simulink model "DeepWaySILForSLX_Trailer_2021a_SteerAngle"  (R2021a)
settings: Solver=FixedStepDiscrete  StartTime=0.0  StopTime=inf  FixedStep=0.001  RelTol=1e-3
InitFcn:
  | TargetIP='10.50.192.52';
libraries: simulink x14, slrealtimeutilitieslib x9, dspnetwork x4, aerolibanimutils x1
(part 1 of 2)
settings Model: Tag=normal  Creator=caowancang  LastModifiedBy=mapen
settings DataIOCC: SaveFormat=StructureWithTime
settings OptimizationCC: DefaultParameterBehavior=Inlined  OptimizeBlockIOStorage=off  EnhancedBackFolding=on  PassReuseOutputArgsAs=Individual arguments  ZeroExternalMemoryAtStartup=off  ZeroInternalMemoryAtStartup=off  OptimizeBlockOrder=speed  DifferentSizesBufferReuse=on  EfficientTunableParamExpr=on
settings DebuggingCC: UnderspecifiedInitializationDetection=Classic  ParameterTunabilityLossMsg=error  FrameProcessingCompatibilityMsg=warning  NonCurrentReleaseOperatingPointMsg=warning
settings SFSimCC: MATLABDynamicMemAlloc=off
settings RTWCC: SystemTargetFile=ert.tlc  TemplateMakefile=ert_default_tmf
settings CodeAppCC: ForceParamTrailComments=on  IgnoreCustomStorageClasses=off  OperatorAnnotations=on  SimulinkDataObjDesc=on  SFDataObjDesc=on  InsertBlockDesc=on
settings ERTTargetCC: TargetLangStandard=C99 (ISO)  GenerateSampleERTMain=on  InlinedParameterPlacement=NonHierarchical  ERTCustomFileTemplate=example_file_process.tlc

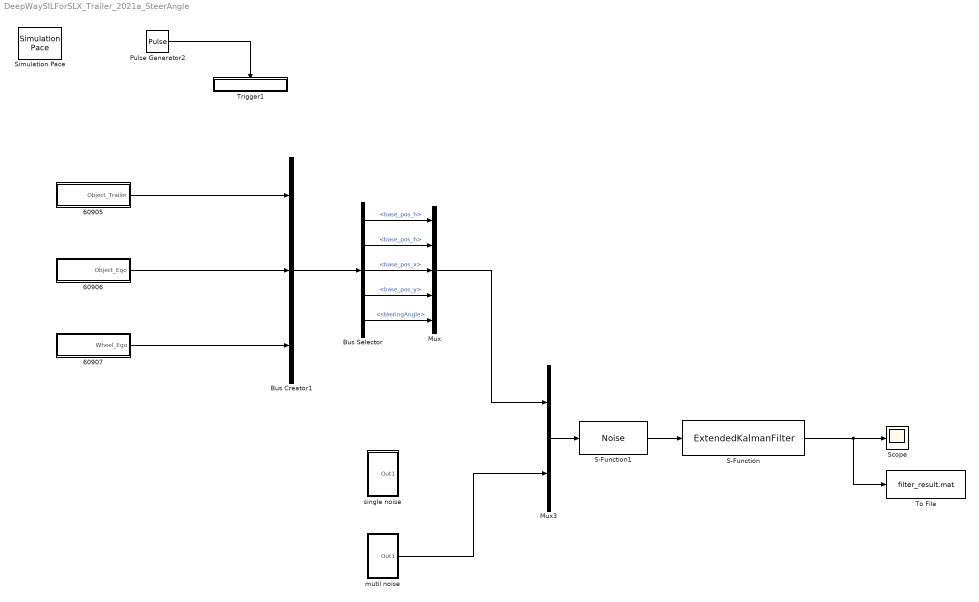
== system DeepWaySILForSLX_Trailer_2021a_SteerAngle ==
  60905 : Subsystem  Description=Modified By caowancang at 2021-11-24 17:03:20.  TreatAsAtomicUnit=on
  60906 : Subsystem  Description=Modified By caowancang at 2021-11-24 17:03:20.  TreatAsAtomicUnit=on
  60907 : Subsystem  Description=Modified By caowancang at 2021-11-24 17:03:20.  TreatAsAtomicUnit=on
  Bus Creator1 : BusCreator  Inputs=3
  Bus Selector : BusSelector  OutputSignals=Object_Ego.Object_Ego.base_pos_h,Object_Trailer.Object_Trailer.base_pos_h,Object_Ego.Object_Ego.base_pos_x,Object_Ego.Object_Ego.base_pos_y,Wheel_Ego.Wheel_Ego.steeringAngle
  Mux : Mux  Inputs=5
  Mux3 : Mux  Inputs=2
  Pulse Generator2 : DiscretePulseGenerator  PulseType=Time based  Period=0.04  PulseWidth=50
  S-Function : S-Function  FunctionName=ExtendedKalmanFilter  SFunctionDeploymentMode=off  EnableBusSupport=off
  S-Function1 : S-Function  FunctionName=Noise  SFunctionDeploymentMode=off  EnableBusSupport=off
  Scope : Scope
  Simulation Pace : aerolibanimutils/Simulation Pace  SimulationPace=1  SleepMode=MATLAB Thread  OutputPaceError=off  SampleTime=-1
      settings: AttributesFormatString=%<SimulationPace> sec/sec
  To File : ToFile  Filename=filter_result.mat  MatrixName=filter_result  SaveFormat=Timeseries
  Trigger1 : Subsystem  Description=Modified By caowancang at 2021-11-26 13:39:19.
  mutil noise : Subsystem
  single noise : Subsystem
  wires:
  60905/1(Object_Trailer) -> Bus Creator1/1
  60906/1(Object_Ego) -> Bus Creator1/2
  Pulse Generator2/1 -> Trigger1/Trigger
  Bus Creator1/1 -> Bus Selector/1
  60907/1(Wheel_Ego) -> Bus Creator1/3
  Bus Selector/1 -> Mux/1  "<base_pos_h>"
  Bus Selector/2 -> Mux/2  "<base_pos_h>"
  Bus Selector/3 -> Mux/3  "<base_pos_x>"
  Bus Selector/4 -> Mux/4  "<base_pos_y>"
  Bus Selector/5 -> Mux/5  "<steeringAngle>"
  Mux/1 -> Mux3/1
  S-Function1/1 -> S-Function/1
  Mux3/1 -> S-Function1/1
  mutil noise/1(Out1) -> Mux3/2
  S-Function/1 -> To File/1, Scope/1

== system DeepWaySILForSLX_Trailer_2021a_SteerAngle/60905 ==
  60905 : Subsystem  Description=Modified By caowancang at 2021-11-18 19:09:14.
  UDP Receive : dspnetwork/UDP Receive  localURL='0.0.0.0'  localPort=60905  remoteURL=TargetIP  remotePort=-1  recvBufferSize=8192  dims=1000  signalDatatype=uint8  isComplex=off  isVarSize=off  showBlockingTime=off  blockingTime=0  sampletime=-1  blockPlatform=[]
  Object_Trailer : Outport  Description=Modified By caowancang at 2021-11-18 18:04:55.
  wires:
  60905/1(Object_Trailer) -> Object_Trailer/1
  UDP Receive/2 -> 60905/2(L)
  UDP Receive/1 -> 60905/1(u)

== system DeepWaySILForSLX_Trailer_2021a_SteerAngle/60906 ==
  60906 : Subsystem  Description=Modified By caowancang at 2021-11-18 19:09:14.
  UDP Receive : dspnetwork/UDP Receive  localURL='0.0.0.0'  localPort=60906  remoteURL=TargetIP  remotePort=-1  recvBufferSize=8192  dims=1000  signalDatatype=uint8  isComplex=off  isVarSize=off  showBlockingTime=off  blockingTime=0  sampletime=-1  blockPlatform=[]
  Object_Ego : Outport  Description=Modified By caowancang at 2021-11-18 18:04:55.
  wires:
  UDP Receive/1 -> 60906/1(u)
  60906/1(Object_Ego) -> Object_Ego/1
  UDP Receive/2 -> 60906/2(L)

== system DeepWaySILForSLX_Trailer_2021a_SteerAngle/60907 ==
  60907 : Subsystem  Description=Modified By caowancang at 2021-11-18 19:09:14.
  UDP Receive : dspnetwork/UDP Receive  localURL='0.0.0.0'  localPort=60907  remoteURL=TargetIP  remotePort=-1  recvBufferSize=8192  dims=1000  signalDatatype=uint8  isComplex=off  isVarSize=off  showBlockingTime=off  blockingTime=0  sampletime=-1  blockPlatform=[]
  Wheel_Ego : Outport  Description=Modified By caowancang at 2021-11-18 18:04:55.
  wires:
  UDP Receive/2 -> 60907/2(L)
  60907/1(Wheel_Ego) -> Wheel_Ego/1
  UDP Receive/1 -> 60907/1(u)

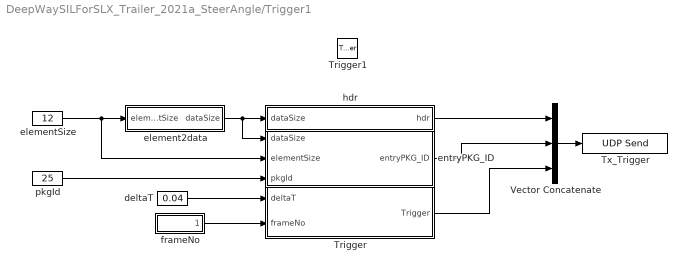
== system DeepWaySILForSLX_Trailer_2021a_SteerAngle/Trigger1 ==
  Trigger1 : TriggerPort  VariantControl=(inherit)
  Trigger : Subsystem  Description=Modified By caowancang at 2021-11-18 02:34:00.
  Tx_Trigger : dspnetwork/UDP Send  remoteURL=TargetIP  remotePort=48191  localURL='0.0.0.0'  localPortSource=Automatically determine  localPort=-1  sendBufferSize=8192  sampletime=-1  blockPlatform=[]  separateLengthPort=0
  Vector Concatenate : Concatenate  NumInputs=3
  deltaT : Constant  Description=Modified By caowancang at 2021-11-29 16:25:47.  Value=0.04
  element2data : Subsystem
  elementSize : Constant  Description=Modified By caowancang at 2021-11-18 02:44:35.  Value=12
  entryPKG_ID : Subsystem  Description=Modified By caowancang at 2021-11-11 11:49:52.
  frameNo : Subsystem
  hdr : Subsystem  Description=Modified By caowancang at 2021-11-11 11:49:52.
  pkgId : Constant  Description=Modified By caowancang at 2021-11-18 02:44:35.  Value=25
  wires:
  entryPKG_ID/1(entryPKG_ID) -> Vector Concatenate/2
  hdr/1(hdr) -> Vector Concatenate/1
  elementSize/1 -> entryPKG_ID/2(elementSize), element2data/1(elementSize)
  element2data/1(dataSize) -> entryPKG_ID/1(dataSize), hdr/1(dataSize)
  Vector Concatenate/1 -> Tx_Trigger/1
  pkgId/1 -> entryPKG_ID/3(pkgId)
  Trigger/1(Trigger) -> Vector Concatenate/3
  deltaT/1 -> Trigger/1(deltaT)
  frameNo/1(frameNo) -> Trigger/2(frameNo)

== system DeepWaySILForSLX_Trailer_2021a_SteerAngle/mutil noise ==
  Mux2 : Mux  Inputs=5
  trailer heading noise : simulink/Sources/Band-Limited White Noise  Cov=[0.05 * 0.05 * 0.1]  Ts=0.1  seed=[23341]
  trator heading noise : simulink/Sources/Band-Limited White Noise  Cov=[0.0 * 0.0 * 0.1]  Ts=0.1  seed=[23341]
  trator steer angle noise : simulink/Sources/Band-Limited White Noise  Cov=[0.00 * 0.00 * 0.1]  Ts=0.1  seed=[23341]
  trator xy noise : simulink/Sources/Band-Limited White Noise  Cov=[0.2 * 0.2 * 0.1]  Ts=0.1  seed=[23341]
  Out1 : Outport
  wires:
  trailer heading noise/1 -> Mux2/2
  trator xy noise/1 -> Mux2/4, Mux2/3
  trator heading noise/1 -> Mux2/1
  Mux2/1 -> Out1/1
  trator steer angle noise/1 -> Mux2/5

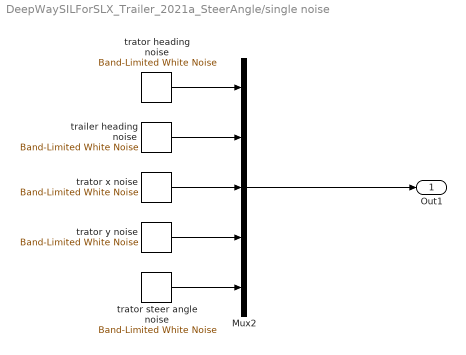
== system DeepWaySILForSLX_Trailer_2021a_SteerAngle/single noise ==
  Mux2 : Mux  Inputs=5
  trailer heading noise : simulink/Sources/Band-Limited White Noise  Cov=[0.05 * 0.05 * 0.1]  Ts=0.1  seed=[23341]
  trator heading noise : simulink/Sources/Band-Limited White Noise  Cov=[0.0 * 0.0 * 0.1]  Ts=0.1  seed=[23341]
  trator steer angle noise : simulink/Sources/Band-Limited White Noise  Cov=[0.0 * 0.0 * 0.1]  Ts=0.1  seed=[23341]
  trator x noise : simulink/Sources/Band-Limited White Noise  Cov=[0.0 * 0.0 * 0.1]  Ts=0.1  seed=[23341]
  trator y noise : simulink/Sources/Band-Limited White Noise  Cov=[0.0 * 0.0 * 0.1]  Ts=0.1  seed=[23341]
  Out1 : Outport
  wires:
  trator y noise/1 -> Mux2/4
  trailer heading noise/1 -> Mux2/2
  trator x noise/1 -> Mux2/3
  trator heading noise/1 -> Mux2/1
  Mux2/1 -> Out1/1
  trator steer angle noise/1 -> Mux2/5

== system DeepWaySILForSLX_Trailer_2021a_SteerAngle/60905/60905 ==
  u : Inport  Description=Modified By caowancang at 2021-11-18 18:43:09.
  L : Inport  Description=Modified By caowancang at 2021-11-18 18:49:26.  Port=2
  98 : Subsystem  Description=Modified By caowancang at 2021-11-18 18:43:09.  TreatAsAtomicUnit=on
  Compare To Constant1 : simulink/Logic and Bit Operations/Compare To Constant  relop===  const=280  OutDataTypeStr=boolean
  Switch Case1 : SwitchCase  CaseConditions={98}  ShowDefaultCase=off
  trigger : Subsystem
  Object_Trailer : Outport  Description=Modified By caowancang at 2021-11-18 18:43:09.
  wires:
  98/1(Object_Trailer) -> Object_Trailer/1
  L/1 -> Compare To Constant1/1
  trigger/1(pkgId) -> Switch Case1/1
  u/1 -> trigger/1(u), 98/1(u)
  Switch Case1/1 -> 98/Action
  Compare To Constant1/1 -> trigger/Trigger

== system DeepWaySILForSLX_Trailer_2021a_SteerAngle/60906/60906 ==
  u : Inport  Description=Modified By caowancang at 2021-11-18 18:43:09.
  L : Inport  Description=Modified By caowancang at 2021-11-18 18:49:26.  Port=2
  97 : Subsystem  Description=Modified By caowancang at 2021-11-18 18:43:09.  TreatAsAtomicUnit=on
  Compare To Constant1 : simulink/Logic and Bit Operations/Compare To Constant  relop===  const=280  OutDataTypeStr=boolean
  Switch Case1 : SwitchCase  CaseConditions={97}  ShowDefaultCase=off
  trigger : Subsystem
  Object_Ego : Outport  Description=Modified By caowancang at 2021-11-18 18:43:09.
  wires:
  97/1(Object_Ego) -> Object_Ego/1
  L/1 -> Compare To Constant1/1
  trigger/1(pkgId) -> Switch Case1/1
  u/1 -> trigger/1(u), 97/1(u)
  Switch Case1/1 -> 97/Action
  Compare To Constant1/1 -> trigger/Trigger

== system DeepWaySILForSLX_Trailer_2021a_SteerAngle/60907/60907 ==
  u : Inport  Description=Modified By caowancang at 2021-11-18 18:43:09.
  L : Inport  Description=Modified By caowancang at 2021-11-18 18:49:26.  Port=2
  99 : Subsystem  Description=Modified By caowancang at 2021-11-18 18:43:09.  TreatAsAtomicUnit=on
  Compare To Constant1 : simulink/Logic and Bit Operations/Compare To Constant  relop===  const=116  OutDataTypeStr=boolean
  Switch Case1 : SwitchCase  CaseConditions={99}  ShowDefaultCase=off
  trigger : Subsystem
  Wheel_Ego : Outport  Description=Modified By caowancang at 2021-11-18 18:43:09.
  wires:
  Compare To Constant1/1 -> trigger/Trigger
  Switch Case1/1 -> 99/Action
  u/1 -> 99/1(u), trigger/1(u)
  trigger/1(pkgId) -> Switch Case1/1
  L/1 -> Compare To Constant1/1
  99/1(Wheel_Ego) -> Wheel_Ego/1

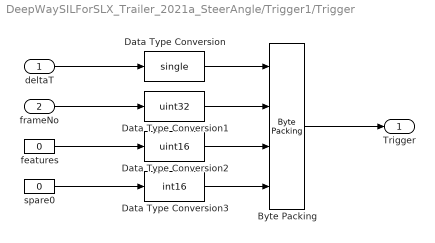
== system DeepWaySILForSLX_Trailer_2021a_SteerAngle/Trigger1/Trigger ==
  deltaT : Inport  Description=Modified By caowancang at 2021-11-18 02:33:49.
  frameNo : Inport  Description=Modified By caowancang at 2021-11-18 02:33:49.  Port=2
  Byte Packing : slrealtimeutilitieslib/Byte Packing  MaskPackedDataType=uint8  MaskUnpackedDataTypes={'single','uint32','uint16','int16'}  MaskAlignment=1
  Data Type Conversion : DataTypeConversion  OutDataTypeStr=single
  Data Type Conversion1 : DataTypeConversion  OutDataTypeStr=uint32
  Data Type Conversion2 : DataTypeConversion  OutDataTypeStr=uint16
  Data Type Conversion3 : DataTypeConversion  OutDataTypeStr=int16
  features : Constant  Description=Modified By caowancang at 2021-11-18 02:33:49.  Value=0
  spare0 : Constant  Description=Modified By caowancang at 2021-11-18 02:33:49.  Value=0
  Trigger : Outport  Description=Modified By caowancang at 2021-11-18 02:33:49.
  wires:
  Data Type Conversion3/1 -> Byte Packing/4
  Data Type Conversion2/1 -> Byte Packing/3
  Data Type Conversion1/1 -> Byte Packing/2
  Data Type Conversion/1 -> Byte Packing/1
  Byte Packing/1 -> Trigger/1
  spare0/1 -> Data Type Conversion3/1
  features/1 -> Data Type Conversion2/1
  frameNo/1 -> Data Type Conversion1/1
  deltaT/1 -> Data Type Conversion/1

== system DeepWaySILForSLX_Trailer_2021a_SteerAngle/Trigger1/element2data ==
  elementSize : Inport  Description=Modified By caowancang at 2021-11-18 02:05:38.
  Constant : Constant  Description=Modified By caowancang at 2021-11-18 02:05:38.
  Product : Product
  dataSize : Outport  Description=Modified By caowancang at 2021-11-18 02:05:38.
  wires:
  Constant/1 -> Product/2
  Product/1 -> dataSize/1
  elementSize/1 -> Product/1

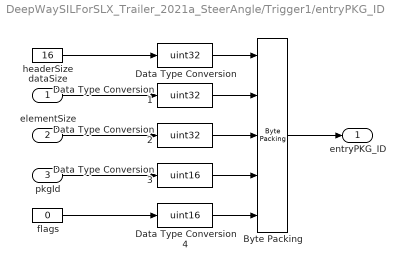
== system DeepWaySILForSLX_Trailer_2021a_SteerAngle/Trigger1/entryPKG_ID ==
  dataSize : Inport  Description=Modified By caowancang at 2021-11-18 02:15:00.
  elementSize : Inport  Description=Modified By caowancang at 2021-11-18 02:15:00.  Port=2
  pkgId : Inport  Description=Modified By caowancang at 2021-11-18 02:15:00.  Port=3
  Byte Packing : slrealtimeutilitieslib/Byte Packing  MaskPackedDataType=uint8  MaskUnpackedDataTypes={'uint32','uint32','uint32','uint16','uint16'}  MaskAlignment=1
  Data Type Conversion : DataTypeConversion  OutDataTypeStr=uint32
  Data Type Conversion1 : DataTypeConversion  OutDataTypeStr=uint32
  Data Type Conversion2 : DataTypeConversion  OutDataTypeStr=uint32
  Data Type Conversion3 : DataTypeConversion  OutDataTypeStr=uint16
  Data Type Conversion4 : DataTypeConversion  OutDataTypeStr=uint16
  flags : Constant  Description=Modified By caowancang at 2021-11-11 11:27:23.  Value=0
  headerSize : Constant  Description=Modified By caowancang at 2021-11-11 11:27:23.  Value=16
  entryPKG_ID : Outport  Description=Modified By caowancang at 2021-11-18 02:24:34.
  wires:
  Data Type Conversion4/1 -> Byte Packing/5
  Data Type Conversion3/1 -> Byte Packing/4
  Data Type Conversion2/1 -> Byte Packing/3
  Data Type Conversion1/1 -> Byte Packing/2
  Data Type Conversion/1 -> Byte Packing/1
  Byte Packing/1 -> entryPKG_ID/1
  headerSize/1 -> Data Type Conversion/1
  dataSize/1 -> Data Type Conversion1/1
  elementSize/1 -> Data Type Conversion2/1
  pkgId/1 -> Data Type Conversion3/1
  flags/1 -> Data Type Conversion4/1

== system DeepWaySILForSLX_Trailer_2021a_SteerAngle/Trigger1/frameNo ==
  Add : Sum
  Compare To Constant : simulink/Logic and Bit Operations/Compare To Constant  relop=>  const=65535  OutDataTypeStr=boolean
  Constant4 : Constant  Description=Modified By caowancang at 2021-11-18 02:07:28.  OutDataTypeStr=uint32
  Switch : Switch  Criteria=u2 ~= 0
  Unit Delay : UnitDelay  SampleTime=-1  HasFrameUpgradeWarning=on
  frameNo : Outport  Description=Modified By caowancang at 2021-11-18 02:07:28.
  wires:
  Compare To Constant/1 -> Switch/2
  Add/1 -> Compare To Constant/1, Switch/3
  Constant4/1 -> Switch/1, Add/1
  Switch/1 -> frameNo/1, Unit Delay/1
  Unit Delay/1 -> Add/2

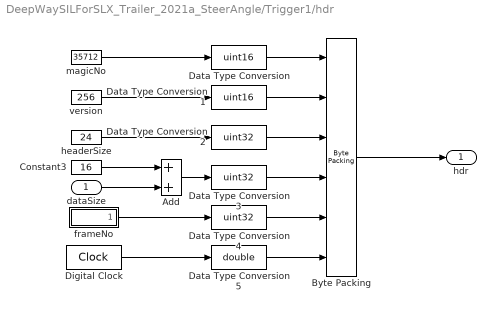
== system DeepWaySILForSLX_Trailer_2021a_SteerAngle/Trigger1/hdr ==
  dataSize : Inport  Description=Modified By caowancang at 2021-11-18 02:12:15.
  Add : Sum
  Byte Packing : slrealtimeutilitieslib/Byte Packing  MaskPackedDataType=uint8  MaskUnpackedDataTypes={'uint16','uint16','uint32','uint32','uint32','double'}  MaskAlignment=1
  Constant3 : Constant  Description=Modified By caowancang at 2021-11-11 11:27:23.  Value=16
  Data Type Conversion : DataTypeConversion  OutDataTypeStr=uint16
  Data Type Conversion1 : DataTypeConversion  OutDataTypeStr=uint16
  Data Type Conversion2 : DataTypeConversion  OutDataTypeStr=uint32
  Data Type Conversion3 : DataTypeConversion  OutDataTypeStr=uint32
  Data Type Conversion4 : DataTypeConversion  OutDataTypeStr=uint32
  Data Type Conversion5 : DataTypeConversion  OutDataTypeStr=double
  Digital Clock : DigitalClock  SampleTime=-1
  frameNo : Subsystem
  headerSize : Constant  Description=Modified By caowancang at 2021-11-11 11:27:23.  Value=24
  magicNo : Constant  Description=Modified By caowancang at 2021-11-11 11:27:23.  Value=35712
  version : Constant  Description=Modified By caowancang at 2021-11-11 11:27:23.  Value=256
  hdr : Outport
  wires:
  Byte Packing/1 -> hdr/1
  Constant3/1 -> Add/1
  Add/1 -> Data Type Conversion3/1
  dataSize/1 -> Add/2
  frameNo/1(frameNo) -> Data Type Conversion4/1
  Digital Clock/1 -> Data Type Conversion5/1
  Data Type Conversion5/1 -> Byte Packing/6
  Data Type Conversion4/1 -> Byte Packing/5
  Data Type Conversion3/1 -> Byte Packing/4
  headerSize/1 -> Data Type Conversion2/1
  Data Type Conversion2/1 -> Byte Packing/3
  version/1 -> Data Type Conversion1/1
  Data Type Conversion1/1 -> Byte Packing/2
  magicNo/1 -> Data Type Conversion/1
  Data Type Conversion/1 -> Byte Packing/1

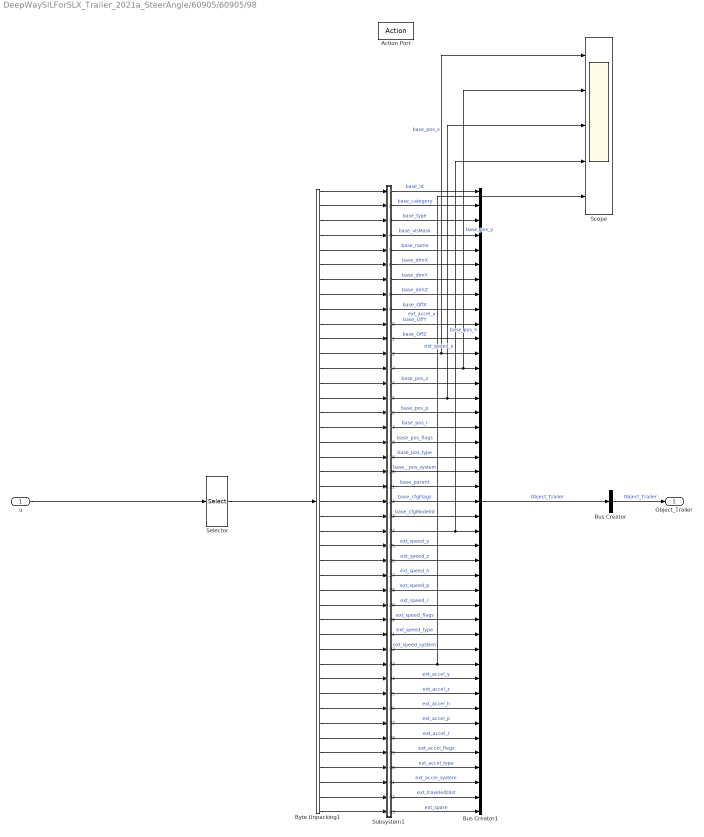
== system DeepWaySILForSLX_Trailer_2021a_SteerAngle/60905/60905/98 ==
  u : Inport  Description=Modified By caowancang at 2021-11-18 14:03:56.
  Action Port : ActionPort  ActionPortLabel=case [ 98 ]:
  Bus Creator : BusCreator  Inputs=1
  Bus Creator1 : BusCreator  Inputs=43
  Byte Unpacking1 : slrealtimeutilitieslib/Byte Unpacking  MaskUnpackedDataTypes={'uint32','uint8','uint8','uint16','uint8','single','single','single','single','single','single','double','double','double','single','single','single','uint8','uint8','uint16','uint32','uint16','int16','double','double','double','single','single','single','uint8','uint8','uint16','double','double','double','single','single','single','uint8','uint8','uint16','single','uint32'}  MaskUnpackedDataSizes={[1],[1],[1],[1],[32],[1],[1],[1],[1],[1],[1],[1],[1],[1],[1],[1],[1],[1],[1],[1],[1],[1],[1],[1],[1],[1],[1],[1],[1],[1],[1],[1],[1],[1],[1],[1],[1],[1],[1],[1],[1],[1],[3]}  MaskAlignment=1
      settings: SourceProductBaseCode=XP
  Scope : Scope  NumInputPorts=5
  Selector : Selector  InputPortWidth=1000  IndexOptions=Starting index (dialog)  Indices=57  OutputSizes=208
  Subsystem1 : Subsystem
  Object_Trailer : Outport  Description=Modified By caowancang at 2021-11-18 14:03:56.
  wires:
  Bus Creator1/1 -> Bus Creator/1  "Object_Trailer"
  Selector/1 -> Byte Unpacking1/1
  u/1 -> Selector/1
  Byte Unpacking1/1 -> Subsystem1/1(In1)
  Byte Unpacking1/2 -> Subsystem1/2(In2)
  Byte Unpacking1/3 -> Subsystem1/3(In3)
  Byte Unpacking1/4 -> Subsystem1/4(In4)
  Byte Unpacking1/5 -> Subsystem1/5(In5)
  Byte Unpacking1/6 -> Subsystem1/6(In6)
  Byte Unpacking1/7 -> Subsystem1/7(In7)
  Byte Unpacking1/8 -> Subsystem1/8(In8)
  Byte Unpacking1/9 -> Subsystem1/9(In9)
  Byte Unpacking1/10 -> Subsystem1/10(In10)
  Byte Unpacking1/11 -> Subsystem1/11(In11)
  Byte Unpacking1/12 -> Subsystem1/12(In12)
  Byte Unpacking1/13 -> Subsystem1/13(In13)
  Byte Unpacking1/14 -> Subsystem1/14(In14)
  Byte Unpacking1/15 -> Subsystem1/15(In15)
  Byte Unpacking1/16 -> Subsystem1/16(In16)
  Byte Unpacking1/17 -> Subsystem1/17(In17)
  Byte Unpacking1/18 -> Subsystem1/18(In18)
  Byte Unpacking1/19 -> Subsystem1/19(In19)
  Byte Unpacking1/20 -> Subsystem1/20(In20)
  Byte Unpacking1/21 -> Subsystem1/21(In21)
  Byte Unpacking1/22 -> Subsystem1/22(In22)
  Byte Unpacking1/23 -> Subsystem1/23(In23)
  Byte Unpacking1/24 -> Subsystem1/24(In24)
  Byte Unpacking1/25 -> Subsystem1/25(In25)
  Byte Unpacking1/26 -> Subsystem1/26(In26)
  Byte Unpacking1/27 -> Subsystem1/27(In27)
  Byte Unpacking1/28 -> Subsystem1/28(In28)
  Byte Unpacking1/29 -> Subsystem1/29(In29)
  Byte Unpacking1/30 -> Subsystem1/30(In30)
  Byte Unpacking1/31 -> Subsystem1/31(In31)
  Byte Unpacking1/32 -> Subsystem1/32(In32)
  Byte Unpacking1/33 -> Subsystem1/33(In33)
  Byte Unpacking1/34 -> Subsystem1/34(In34)
  Byte Unpacking1/35 -> Subsystem1/35(In35)
  Byte Unpacking1/36 -> Subsystem1/36(In36)
  Byte Unpacking1/37 -> Subsystem1/37(In37)
  Byte Unpacking1/38 -> Subsystem1/38(In38)
  Byte Unpacking1/39 -> Subsystem1/39(In39)
  Byte Unpacking1/40 -> Subsystem1/40(In40)
  Byte Unpacking1/41 -> Subsystem1/41(In41)
  Byte Unpacking1/42 -> Subsystem1/42(In42)
  Byte Unpacking1/43 -> Subsystem1/43(In43)
  Subsystem1/1(base_id) -> Bus Creator1/1  "base_id"
  Subsystem1/2(category) -> Bus Creator1/2  "base_category"
  Subsystem1/3(type) -> Bus Creator1/3  "base_type"
  Subsystem1/4(visMask) -> Bus Creator1/4  "base_visMask"
  Subsystem1/5(name) -> Bus Creator1/5  "base_name"
  Subsystem1/6(dimX) -> Bus Creator1/6  "base_dimX"
  Subsystem1/7(dimY) -> Bus Creator1/7  "base_dimY"
  Subsystem1/8(dimZ) -> Bus Creator1/8  "base_dimZ"
  Subsystem1/9(OffX) -> Bus Creator1/9  "base_OffX"
  Subsystem1/10(OffY) -> Bus Creator1/10  "base_OffY"
  Subsystem1/11(OffZ) -> Bus Creator1/11  "base_OffZ"
  Subsystem1/12(pos_x) -> Scope/1, Bus Creator1/12  "base_pos_x"
  Subsystem1/13(pos_y) -> Scope/2, Bus Creator1/13  "base_pos_y"
  Subsystem1/14(pos_z) -> Bus Creator1/14  "base_pos_z"
  Subsystem1/15(pos_h) -> Scope/3, Bus Creator1/15  "base_pos_h"
  Subsystem1/16(pos_p) -> Bus Creator1/16  "base_pos_p"
  Subsystem1/17(pos_r) -> Bus Creator1/17  "base_pos_r"
  Subsystem1/18(flags) -> Bus Creator1/18  "base_pos_flags"
  Subsystem1/19(type1) -> Bus Creator1/19  "base_pos_type"
  Subsystem1/20(system) -> Bus Creator1/20  "base__pos_system"
  Subsystem1/21(parent) -> Bus Creator1/21  "base_parent"
  Subsystem1/22(cfgFlags) -> Bus Creator1/22  "base_cfgFlags"
  Subsystem1/23(cfgModelId) -> Bus Creator1/23  "base_cfgModelId"
  Subsystem1/24(speed_x) -> Scope/4, Bus Creator1/24  "ext_speed_x"
  Subsystem1/25(speed_y) -> Bus Creator1/25  "ext_speed_y"
  Subsystem1/26(speed_z) -> Bus Creator1/26  "ext_speed_z"
  Subsystem1/27(speed_h) -> Bus Creator1/27  "ext_speed_h"
  Subsystem1/28(speed_p) -> Bus Creator1/28  "ext_speed_p"
  Subsystem1/29(speed_r) -> Bus Creator1/29  "ext_speed_r"
  Subsystem1/30(flags2) -> Bus Creator1/30  "ext_speed_flags"
  Subsystem1/31(type3) -> Bus Creator1/31  "ext_speed_type"
  Subsystem1/32(system2) -> Bus Creator1/32  "ext_speed_system"
  Subsystem1/33(accel_x) -> Scope/5, Bus Creator1/33  "ext_accel_x"
  Subsystem1/34(accel_y) -> Bus Creator1/34  "ext_accel_y"
  Subsystem1/35(accel_z) -> Bus Creator1/35  "ext_accel_z"
  Subsystem1/36(accel_h) -> Bus Creator1/36  "ext_accel_h"
  Subsystem1/37(accel_p) -> Bus Creator1/37  "ext_accel_p"
  Subsystem1/38(accel_r) -> Bus Creator1/38  "ext_accel_r"
  Subsystem1/39(flags1) -> Bus Creator1/39  "ext_accel_flags"
  Subsystem1/40(type2) -> Bus Creator1/40  "ext_accel_type"
  Subsystem1/41(system1) -> Bus Creator1/41  "ext_accel_system"
  Subsystem1/42(traveledDist) -> Bus Creator1/42  "ext_traveledDist"
  Subsystem1/43(spare_1) -> Bus Creator1/43  "ext_spare"
  Bus Creator/1 -> Object_Trailer/1  "Object_Trailer"

== system DeepWaySILForSLX_Trailer_2021a_SteerAngle/60905/60905/trigger ==
  u : Inport  Description=Modified By caowancang at 2021-11-18 18:42:51.
  Trigger : TriggerPort  VariantControl=(inherit)
  Byte Unpacking : slrealtimeutilitieslib/Byte Unpacking  MaskUnpackedDataTypes={'uint16'}  MaskUnpackedDataSizes={[1]}  MaskAlignment=1
      settings: SourceProductBaseCode=XP
  Selector : Selector  InputPortWidth=1000  IndexOptions=Starting index (dialog)  Indices=53  OutputSizes=2
  pkgId : Outport  Description=Modified By caowancang at 2021-11-18 18:42:51.
  wires:
  Selector/1 -> Byte Unpacking/1
  u/1 -> Selector/1
  Byte Unpacking/1 -> pkgId/1  "pkgId"

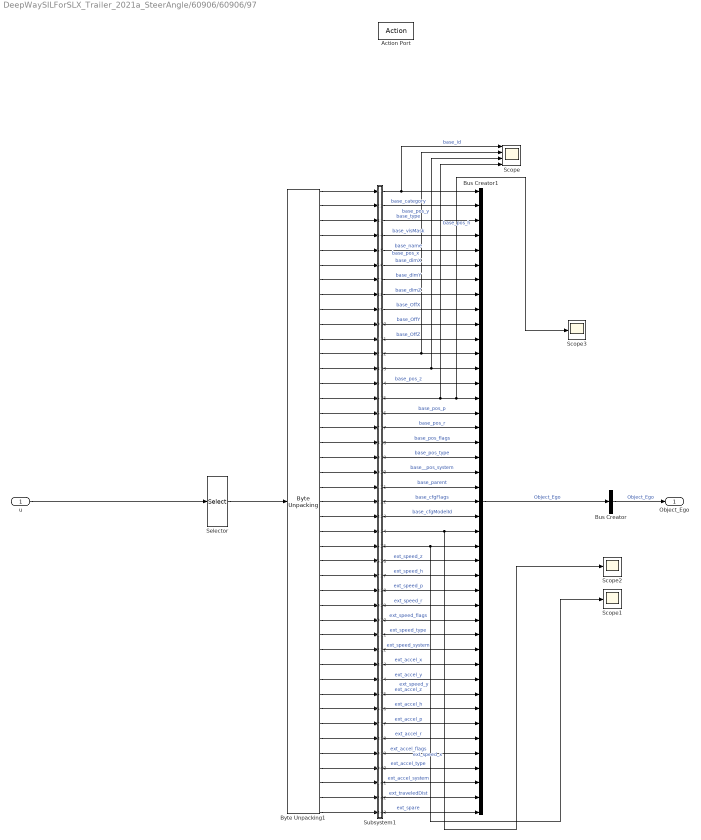
== system DeepWaySILForSLX_Trailer_2021a_SteerAngle/60906/60906/97 ==
  u : Inport  Description=Modified By caowancang at 2021-11-18 14:03:56.
  Action Port : ActionPort  ActionPortLabel=case [ 97 ]:
  Bus Creator : BusCreator  Inputs=1
  Bus Creator1 : BusCreator  Inputs=43
  Byte Unpacking1 : slrealtimeutilitieslib/Byte Unpacking  MaskUnpackedDataTypes={'uint32','uint8','uint8','uint16','uint8','single','single','single','single','single','single','double','double','double','single','single','single','uint8','uint8','uint16','uint32','uint16','int16','double','double','double','single','single','single','uint8','uint8','uint16','double','double','double','single','single','single','uint8','uint8','uint16','single','uint32'}  MaskUnpackedDataSizes={[1],[1],[1],[1],[32],[1],[1],[1],[1],[1],[1],[1],[1],[1],[1],[1],[1],[1],[1],[1],[1],[1],[1],[1],[1],[1],[1],[1],[1],[1],[1],[1],[1],[1],[1],[1],[1],[1],[1],[1],[1],[1],[3]}  MaskAlignment=1
      settings: SourceProductBaseCode=XP
  Scope : Scope  NumInputPorts=4
  Scope1 : Scope
  Scope2 : Scope
  Scope3 : Scope
  Selector : Selector  InputPortWidth=1000  IndexOptions=Starting index (dialog)  Indices=57  OutputSizes=208
  Subsystem1 : Subsystem
  Object_Ego : Outport  Description=Modified By caowancang at 2021-11-18 14:03:56.
  wires:
  Bus Creator1/1 -> Bus Creator/1  "Object_Ego"
  Selector/1 -> Byte Unpacking1/1
  u/1 -> Selector/1
  Byte Unpacking1/1 -> Subsystem1/1(In1)
  Byte Unpacking1/2 -> Subsystem1/2(In2)
  Byte Unpacking1/3 -> Subsystem1/3(In3)
  Byte Unpacking1/4 -> Subsystem1/4(In4)
  Byte Unpacking1/5 -> Subsystem1/5(In5)
  Byte Unpacking1/6 -> Subsystem1/6(In6)
  Byte Unpacking1/7 -> Subsystem1/7(In7)
  Byte Unpacking1/8 -> Subsystem1/8(In8)
  Byte Unpacking1/9 -> Subsystem1/9(In9)
  Byte Unpacking1/10 -> Subsystem1/10(In10)
  Byte Unpacking1/11 -> Subsystem1/11(In11)
  Byte Unpacking1/12 -> Subsystem1/12(In12)
  Byte Unpacking1/13 -> Subsystem1/13(In13)
  Byte Unpacking1/14 -> Subsystem1/14(In14)
  Byte Unpacking1/15 -> Subsystem1/15(In15)
  Byte Unpacking1/16 -> Subsystem1/16(In16)
  Byte Unpacking1/17 -> Subsystem1/17(In17)
  Byte Unpacking1/18 -> Subsystem1/18(In18)
  Byte Unpacking1/19 -> Subsystem1/19(In19)
  Byte Unpacking1/20 -> Subsystem1/20(In20)
  Byte Unpacking1/21 -> Subsystem1/21(In21)
  Byte Unpacking1/22 -> Subsystem1/22(In22)
  Byte Unpacking1/23 -> Subsystem1/23(In23)
  Byte Unpacking1/24 -> Subsystem1/24(In24)
  Byte Unpacking1/25 -> Subsystem1/25(In25)
  Byte Unpacking1/26 -> Subsystem1/26(In26)
  Byte Unpacking1/27 -> Subsystem1/27(In27)
  Byte Unpacking1/28 -> Subsystem1/28(In28)
  Byte Unpacking1/29 -> Subsystem1/29(In29)
  Byte Unpacking1/30 -> Subsystem1/30(In30)
  Byte Unpacking1/31 -> Subsystem1/31(In31)
  Byte Unpacking1/32 -> Subsystem1/32(In32)
  Byte Unpacking1/33 -> Subsystem1/33(In33)
  Byte Unpacking1/34 -> Subsystem1/34(In34)
  Byte Unpacking1/35 -> Subsystem1/35(In35)
  Byte Unpacking1/36 -> Subsystem1/36(In36)
  Byte Unpacking1/37 -> Subsystem1/37(In37)
  Byte Unpacking1/38 -> Subsystem1/38(In38)
  Byte Unpacking1/39 -> Subsystem1/39(In39)
  Byte Unpacking1/40 -> Subsystem1/40(In40)
  Byte Unpacking1/41 -> Subsystem1/41(In41)
  Byte Unpacking1/42 -> Subsystem1/42(In42)
  Byte Unpacking1/43 -> Subsystem1/43(In43)
  Subsystem1/1(base_id) -> Scope/1, Bus Creator1/1  "base_id"
  Subsystem1/2(category) -> Bus Creator1/2  "base_category"
  Subsystem1/3(type) -> Bus Creator1/3  "base_type"
  Subsystem1/4(visMask) -> Bus Creator1/4  "base_visMask"
  Subsystem1/5(name) -> Bus Creator1/5  "base_name"
  Subsystem1/6(dimX) -> Bus Creator1/6  "base_dimX"
  Subsystem1/7(dimY) -> Bus Creator1/7  "base_dimY"
  Subsystem1/8(dimZ) -> Bus Creator1/8  "base_dimZ"
  Subsystem1/9(OffX) -> Bus Creator1/9  "base_OffX"
  Subsystem1/10(OffY) -> Bus Creator1/10  "base_OffY"
  Subsystem1/11(OffZ) -> Bus Creator1/11  "base_OffZ"
  Subsystem1/12(pos_x) -> Bus Creator1/12, Scope/2  "base_pos_x"
  Subsystem1/13(pos_y) -> Scope/3, Bus Creator1/13  "base_pos_y"
  Subsystem1/14(pos_z) -> Bus Creator1/14  "base_pos_z"
  Subsystem1/15(pos_h) -> Scope/4, Scope3/1, Bus Creator1/15  "base_pos_h"
  Subsystem1/16(pos_p) -> Bus Creator1/16  "base_pos_p"
  Subsystem1/17(pos_r) -> Bus Creator1/17  "base_pos_r"
  Subsystem1/18(flags) -> Bus Creator1/18  "base_pos_flags"
  Subsystem1/19(type1) -> Bus Creator1/19  "base_pos_type"
  Subsystem1/20(system) -> Bus Creator1/20  "base__pos_system"
  Subsystem1/21(parent) -> Bus Creator1/21  "base_parent"
  Subsystem1/22(cfgFlags) -> Bus Creator1/22  "base_cfgFlags"
  Subsystem1/23(cfgModelId) -> Bus Creator1/23  "base_cfgModelId"
  Subsystem1/24(speed_x) -> Scope2/1, Bus Creator1/24  "ext_speed_x"
  Subsystem1/25(speed_y) -> Scope1/1, Bus Creator1/25  "ext_speed_y"
  Subsystem1/26(speed_z) -> Bus Creator1/26  "ext_speed_z"
  Subsystem1/27(speed_h) -> Bus Creator1/27  "ext_speed_h"
  Subsystem1/28(speed_p) -> Bus Creator1/28  "ext_speed_p"
  Subsystem1/29(speed_r) -> Bus Creator1/29  "ext_speed_r"
  Subsystem1/30(flags2) -> Bus Creator1/30  "ext_speed_flags"
  Subsystem1/31(type3) -> Bus Creator1/31  "ext_speed_type"
  Subsystem1/32(system2) -> Bus Creator1/32  "ext_speed_system"
  Subsystem1/33(accel_x) -> Bus Creator1/33  "ext_accel_x"
  Subsystem1/34(accel_y) -> Bus Creator1/34  "ext_accel_y"
  Subsystem1/35(accel_z) -> Bus Creator1/35  "ext_accel_z"
  Subsystem1/36(accel_h) -> Bus Creator1/36  "ext_accel_h"
  Subsystem1/37(accel_p) -> Bus Creator1/37  "ext_accel_p"
  Subsystem1/38(accel_r) -> Bus Creator1/38  "ext_accel_r"
  Subsystem1/39(flags1) -> Bus Creator1/39  "ext_accel_flags"
  Subsystem1/40(type2) -> Bus Creator1/40  "ext_accel_type"
  Subsystem1/41(system1) -> Bus Creator1/41  "ext_accel_system"
  Subsystem1/42(traveledDist) -> Bus Creator1/42  "ext_traveledDist"
  Subsystem1/43(spare_1) -> Bus Creator1/43  "ext_spare"
  Bus Creator/1 -> Object_Ego/1  "Object_Ego"

== system DeepWaySILForSLX_Trailer_2021a_SteerAngle/60906/60906/trigger ==
  u : Inport  Description=Modified By caowancang at 2021-11-18 18:42:51.
  Trigger : TriggerPort  VariantControl=(inherit)
  Byte Unpacking : slrealtimeutilitieslib/Byte Unpacking  MaskUnpackedDataTypes={'uint16'}  MaskUnpackedDataSizes={[1]}  MaskAlignment=1
      settings: SourceProductBaseCode=XP
  Selector : Selector  InputPortWidth=1000  IndexOptions=Starting index (dialog)  Indices=53  OutputSizes=2
  pkgId : Outport  Description=Modified By caowancang at 2021-11-18 18:42:51.
  wires:
  Selector/1 -> Byte Unpacking/1
  u/1 -> Selector/1
  Byte Unpacking/1 -> pkgId/1  "pkgId"

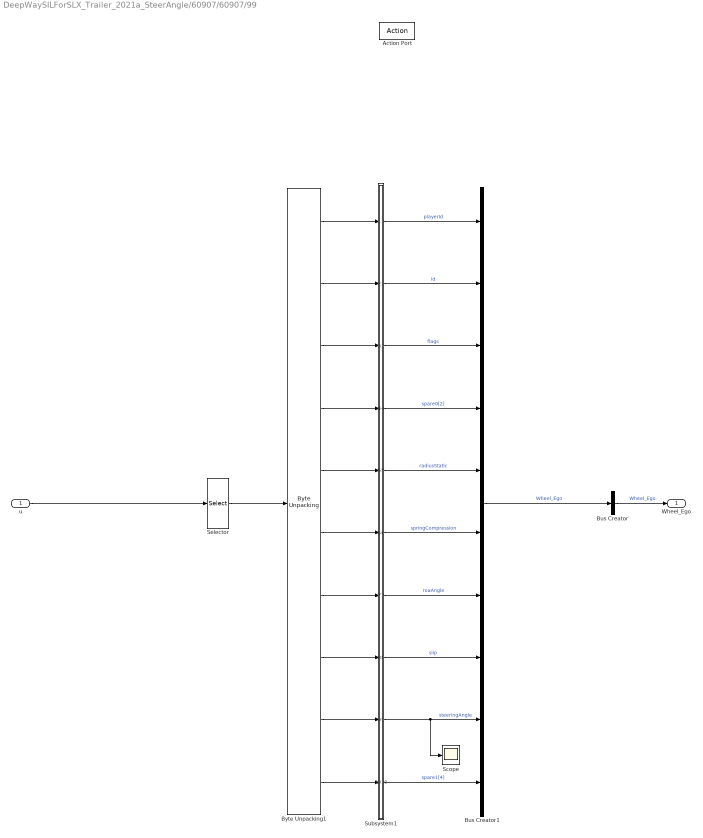
== system DeepWaySILForSLX_Trailer_2021a_SteerAngle/60907/60907/99 ==
  u : Inport  Description=Modified By caowancang at 2021-11-18 14:03:56.
  Action Port : ActionPort  ActionPortLabel=case [ 99 ]:
  Bus Creator : BusCreator  Inputs=1
  Bus Creator1 : BusCreator  Inputs=10
  Byte Unpacking1 : slrealtimeutilitieslib/Byte Unpacking  MaskUnpackedDataTypes={'uint32','uint8','uint8','uint8','single','single','single','single','single','uint32'}  MaskUnpackedDataSizes={[1],[1],[1],[2],[1],[1],[1],[1],[1],[4]}  MaskAlignment=1
      settings: SourceProductBaseCode=XP
  Scope : Scope
  Selector : Selector  InputPortWidth=1000  IndexOptions=Starting index (dialog)  Indices=57  OutputSizes=44
  Subsystem1 : Subsystem
  Wheel_Ego : Outport  Description=Modified By caowancang at 2021-11-18 14:03:56.
  wires:
  Bus Creator/1 -> Wheel_Ego/1  "Wheel_Ego"
  u/1 -> Selector/1
  Selector/1 -> Byte Unpacking1/1
  Bus Creator1/1 -> Bus Creator/1  "Wheel_Ego"
  Byte Unpacking1/1 -> Subsystem1/1(In1)
  Byte Unpacking1/2 -> Subsystem1/2(In2)
  Byte Unpacking1/3 -> Subsystem1/3(In3)
  Byte Unpacking1/4 -> Subsystem1/4(In4)
  Byte Unpacking1/5 -> Subsystem1/5(In5)
  Byte Unpacking1/6 -> Subsystem1/6(In6)
  Byte Unpacking1/7 -> Subsystem1/7(In7)
  Byte Unpacking1/8 -> Subsystem1/8(In8)
  Byte Unpacking1/9 -> Subsystem1/9(In9)
  Byte Unpacking1/10 -> Subsystem1/10(In10)
  Subsystem1/1(base_id) -> Bus Creator1/1  "playerId"
  Subsystem1/2(category) -> Bus Creator1/2  "id"
  Subsystem1/3(type) -> Bus Creator1/3  "flags"
  Subsystem1/4(visMask) -> Bus Creator1/4  "spare0[2]"
  Subsystem1/5(name) -> Bus Creator1/5  "radiusStatic"
  Subsystem1/6(dimX) -> Bus Creator1/6  "springCompression"
  Subsystem1/7(dimY) -> Bus Creator1/7  "roaAngle"
  Subsystem1/8(dimZ) -> Bus Creator1/8  "slip"
  Subsystem1/9(OffX) -> Scope/1, Bus Creator1/9  "steeringAngle"
  Subsystem1/10(OffY) -> Bus Creator1/10  "spare1[4]"

== system DeepWaySILForSLX_Trailer_2021a_SteerAngle/60907/60907/trigger ==
  u : Inport  Description=Modified By caowancang at 2021-11-18 18:42:51.
  Trigger : TriggerPort  VariantControl=(inherit)
  Byte Unpacking : slrealtimeutilitieslib/Byte Unpacking  MaskUnpackedDataTypes={'uint16'}  MaskUnpackedDataSizes={[1]}  MaskAlignment=1
      settings: SourceProductBaseCode=XP
  Selector : Selector  InputPortWidth=1000  IndexOptions=Starting index (dialog)  Indices=53  OutputSizes=2
  pkgId : Outport  Description=Modified By caowancang at 2021-11-18 18:42:51.
  wires:
  Byte Unpacking/1 -> pkgId/1  "pkgId"
  u/1 -> Selector/1
  Selector/1 -> Byte Unpacking/1

== system DeepWaySILForSLX_Trailer_2021a_SteerAngle/Trigger1/hdr/frameNo ==
  Add : Sum
  Compare To Constant : simulink/Logic and Bit Operations/Compare To Constant  relop=>  const=65535  OutDataTypeStr=boolean
  Constant4 : Constant  Description=Modified By caowancang at 2021-11-18 02:07:28.  OutDataTypeStr=uint32
  Switch : Switch  Criteria=u2 ~= 0
  Unit Delay : UnitDelay  SampleTime=-1  HasFrameUpgradeWarning=on
  frameNo : Outport  Description=Modified By caowancang at 2021-11-18 02:07:28.
  wires:
  Compare To Constant/1 -> Switch/2
  Add/1 -> Compare To Constant/1, Switch/3
  Constant4/1 -> Switch/1, Add/1
  Switch/1 -> frameNo/1, Unit Delay/1
  Unit Delay/1 -> Add/2

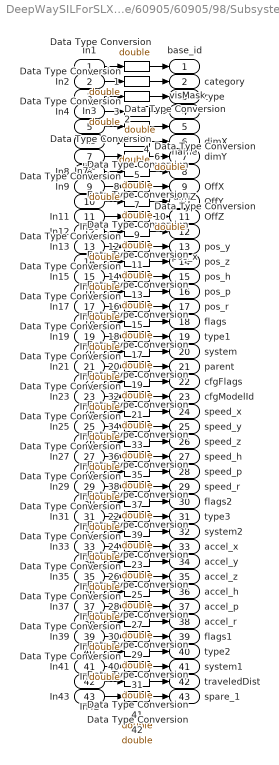
== system DeepWaySILForSLX_Trailer_2021a_SteerAngle/60905/60905/98/Subsystem1 ==
  In1 : Inport  Description=Modified By caowancang at 2021-11-19 16:04:52.
  In2 : Inport  Description=Modified By caowancang at 2021-11-19 16:04:52.  Port=2
  In3 : Inport  Description=Modified By caowancang at 2021-11-19 16:04:52.  Port=3
  In4 : Inport  Description=Modified By caowancang at 2021-11-19 16:04:52.  Port=4
  In5 : Inport  Description=Modified By caowancang at 2021-11-19 16:04:52.  Port=5
  In6 : Inport  Description=Modified By caowancang at 2021-11-19 16:04:52.  Port=6
  In7 : Inport  Description=Modified By caowancang at 2021-11-19 16:04:52.  Port=7
  In8 : Inport  Description=Modified By caowancang at 2021-11-19 16:04:52.  Port=8
  In9 : Inport  Description=Modified By caowancang at 2021-11-19 16:04:52.  Port=9
  In10 : Inport  Description=Modified By caowancang at 2021-11-19 16:04:52.  Port=10
  In11 : Inport  Description=Modified By caowancang at 2021-11-19 16:04:52.  Port=11
  In12 : Inport  Description=Modified By caowancang at 2021-11-19 16:04:52.  Port=12
  In13 : Inport  Description=Modified By caowancang at 2021-11-19 16:04:52.  Port=13
  In14 : Inport  Description=Modified By caowancang at 2021-11-19 16:04:52.  Port=14
  In15 : Inport  Description=Modified By caowancang at 2021-11-19 16:04:52.  Port=15
  In16 : Inport  Description=Modified By caowancang at 2021-11-19 16:04:52.  Port=16
  In17 : Inport  Description=Modified By caowancang at 2021-11-19 16:04:52.  Port=17
  In18 : Inport  Description=Modified By caowancang at 2021-11-19 16:04:52.  Port=18
  In19 : Inport  Description=Modified By caowancang at 2021-11-19 16:04:52.  Port=19
  In20 : Inport  Description=Modified By caowancang at 2021-11-19 16:04:52.  Port=20
  In21 : Inport  Description=Modified By caowancang at 2021-11-19 16:04:52.  Port=21
  In22 : Inport  Description=Modified By caowancang at 2021-11-19 16:04:52.  Port=22
  In23 : Inport  Description=Modified By caowancang at 2021-11-19 16:04:52.  Port=23
  In24 : Inport  Description=Modified By caowancang at 2021-11-19 16:04:52.  Port=24
  In25 : Inport  Description=Modified By caowancang at 2021-11-19 16:04:52.  Port=25
  In26 : Inport  Description=Modified By caowancang at 2021-11-19 16:04:52.  Port=26
  In27 : Inport  Description=Modified By caowancang at 2021-11-19 16:04:52.  Port=27
  In28 : Inport  Description=Modified By caowancang at 2021-11-19 16:04:52.  Port=28
  In29 : Inport  Description=Modified By caowancang at 2021-11-19 16:04:52.  Port=29
  In30 : Inport  Description=Modified By caowancang at 2021-11-19 16:04:52.  Port=30
  In31 : Inport  Description=Modified By caowancang at 2021-11-19 16:04:52.  Port=31
  In32 : Inport  Description=Modified By caowancang at 2021-11-19 16:04:52.  Port=32
  In33 : Inport  Description=Modified By caowancang at 2021-11-19 16:04:52.  Port=33
  In34 : Inport  Description=Modified By caowancang at 2021-11-19 16:04:52.  Port=34
  In35 : Inport  Description=Modified By caowancang at 2021-11-19 16:04:52.  Port=35
  In36 : Inport  Description=Modified By caowancang at 2021-11-19 16:04:52.  Port=36
  In37 : Inport  Description=Modified By caowancang at 2021-11-19 16:04:52.  Port=37
  In38 : Inport  Description=Modified By caowancang at 2021-11-19 16:04:52.  Port=38
  In39 : Inport  Description=Modified By caowancang at 2021-11-19 16:04:52.  Port=39
  In40 : Inport  Description=Modified By caowancang at 2021-11-19 16:04:52.  Port=40
  In41 : Inport  Description=Modified By caowancang at 2021-11-19 16:04:52.  Port=41
  In42 : Inport  Description=Modified By caowancang at 2021-11-19 16:04:52.  Port=42
  In43 : Inport  Description=Modified By caowancang at 2021-11-19 16:04:52.  Port=43
  Data Type Conversion{,1..42} (43 alike) : DataTypeConversion  OutDataTypeStr=double
  base_id : Outport  Description=Modified By caowancang at 2021-11-19 16:04:52.
  category : Outport  Description=Modified By caowancang at 2021-11-19 16:04:52.  Port=2
  type : Outport  Description=Modified By caowancang at 2021-11-19 16:04:52.  Port=3
  visMask : Outport  Description=Modified By caowancang at 2021-11-19 16:04:52.  Port=4
  name : Outport  Description=Modified By caowancang at 2021-11-19 16:04:52.  Port=5
  dimX : Outport  Description=Modified By caowancang at 2021-11-19 16:04:52.  Port=6
  dimY : Outport  Description=Modified By caowancang at 2021-11-19 16:04:52.  Port=7
  dimZ : Outport  Description=Modified By caowancang at 2021-11-19 16:04:52.  Port=8
  OffX : Outport  Description=Modified By caowancang at 2021-11-19 16:04:52.  Port=9
  OffY : Outport  Description=Modified By caowancang at 2021-11-19 16:04:52.  Port=10
  OffZ : Outport  Description=Modified By caowancang at 2021-11-19 16:04:52.  Port=11
  pos_x : Outport  Description=Modified By caowancang at 2021-11-19 16:04:52.  Port=12
  pos_y : Outport  Description=Modified By caowancang at 2021-11-19 16:04:52.  Port=13
  pos_z : Outport  Description=Modified By caowancang at 2021-11-19 16:04:52.  Port=14
  pos_h : Outport  Description=Modified By caowancang at 2021-11-19 16:04:52.  Port=15
  pos_p : Outport  Description=Modified By caowancang at 2021-11-19 16:04:52.  Port=16
  pos_r : Outport  Description=Modified By caowancang at 2021-11-19 16:04:52.  Port=17
  flags : Outport  Description=Modified By caowancang at 2021-11-19 16:04:52.  Port=18
  type1 : Outport  Description=Modified By caowancang at 2021-11-19 16:04:52.  Port=19
  system : Outport  Description=Modified By caowancang at 2021-11-19 16:04:52.  Port=20
  parent : Outport  Description=Modified By caowancang at 2021-11-19 16:04:52.  Port=21
  cfgFlags : Outport  Description=Modified By caowancang at 2021-11-19 16:04:52.  Port=22
  cfgModelId : Outport  Description=Modified By caowancang at 2021-11-19 16:04:52.  Port=23
  speed_x : Outport  Description=Modified By caowancang at 2021-11-19 16:04:52.  Port=24
  speed_y : Outport  Description=Modified By caowancang at 2021-11-19 16:04:52.  Port=25
  speed_z : Outport  Description=Modified By caowancang at 2021-11-19 16:04:52.  Port=26
  speed_h : Outport  Description=Modified By caowancang at 2021-11-19 16:04:52.  Port=27
  speed_p : Outport  Description=Modified By caowancang at 2021-11-19 16:04:52.  Port=28
  speed_r : Outport  Description=Modified By caowancang at 2021-11-19 16:04:52.  Port=29
  flags2 : Outport  Description=Modified By caowancang at 2021-11-19 16:04:52.  Port=30
  type3 : Outport  Description=Modified By caowancang at 2021-11-19 16:04:52.  Port=31
  system2 : Outport  Description=Modified By caowancang at 2021-11-19 16:04:52.  Port=32
  accel_x : Outport  Description=Modified By caowancang at 2021-11-19 16:04:52.  Port=33
  accel_y : Outport  Description=Modified By caowancang at 2021-11-19 16:04:52.  Port=34
  accel_z : Outport  Description=Modified By caowancang at 2021-11-19 16:04:52.  Port=35
  accel_h : Outport  Description=Modified By caowancang at 2021-11-19 16:04:52.  Port=36
  accel_p : Outport  Description=Modified By caowancang at 2021-11-19 16:04:52.  Port=37
  accel_r : Outport  Description=Modified By caowancang at 2021-11-19 16:04:52.  Port=38
  flags1 : Outport  Description=Modified By caowancang at 2021-11-19 16:04:52.  Port=39
  type2 : Outport  Description=Modified By caowancang at 2021-11-19 16:04:52.  Port=40
  system1 : Outport  Description=Modified By caowancang at 2021-11-19 16:04:52.  Port=41
  traveledDist : Outport  Description=Modified By caowancang at 2021-11-19 16:04:52.  Port=42
  spare_1 : Outport  Description=Modified By caowancang at 2021-11-19 16:04:52.  Port=43
  wires:
  In4/1 -> Data Type Conversion3/1
  Data Type Conversion3/1 -> visMask/1
  Data Type Conversion2/1 -> type/1
  In3/1 -> Data Type Conversion2/1
  In2/1 -> Data Type Conversion1/1
  Data Type Conversion1/1 -> category/1
  Data Type Conversion/1 -> base_id/1
  In1/1 -> Data Type Conversion/1
  Data Type Conversion4/1 -> name/1
  In5/1 -> Data Type Conversion4/1
  In10/1 -> Data Type Conversion9/1
  Data Type Conversion9/1 -> OffY/1
  In6/1 -> Data Type Conversion5/1
  Data Type Conversion5/1 -> dimX/1
  Data Type Conversion6/1 -> dimY/1
  In7/1 -> Data Type Conversion6/1
  In8/1 -> Data Type Conversion7/1
  Data Type Conversion7/1 -> dimZ/1
  Data Type Conversion8/1 -> OffX/1
  In9/1 -> Data Type Conversion8/1
  In19/1 -> Data Type Conversion18/1
  Data Type Conversion18/1 -> type1/1
  Data Type Conversion17/1 -> flags/1
  In18/1 -> Data Type Conversion17/1
  In17/1 -> Data Type Conversion16/1
  Data Type Conversion16/1 -> pos_r/1
  Data Type Conversion15/1 -> pos_p/1
  In16/1 -> Data Type Conversion15/1
  Data Type Conversion19/1 -> system/1
  In20/1 -> Data Type Conversion19/1
  In15/1 -> Data Type Conversion14/1
  Data Type Conversion14/1 -> pos_h/1
  In11/1 -> Data Type Conversion10/1
  Data Type Conversion10/1 -> OffZ/1
  Data Type Conversion11/1 -> pos_x/1
  In12/1 -> Data Type Conversion11/1
  In13/1 -> Data Type Conversion12/1
  Data Type Conversion12/1 -> pos_y/1
  Data Type Conversion13/1 -> pos_z/1
  In14/1 -> Data Type Conversion13/1
  In34/1 -> Data Type Conversion25/1
  Data Type Conversion25/1 -> accel_y/1
  Data Type Conversion24/1 -> accel_x/1
  In33/1 -> Data Type Conversion24/1
  In32/1 -> Data Type Conversion23/1
  Data Type Conversion23/1 -> system2/1
  Data Type Conversion22/1 -> type3/1
  In31/1 -> Data Type Conversion22/1
  Data Type Conversion26/1 -> accel_z/1
  In35/1 -> Data Type Conversion26/1
  In40/1 -> Data Type Conversion31/1
  Data Type Conversion31/1 -> type2/1
  In36/1 -> Data Type Conversion27/1
  Data Type Conversion27/1 -> accel_h/1
  Data Type Conversion28/1 -> accel_p/1
  In37/1 -> Data Type Conversion28/1
  In38/1 -> Data Type Conversion29/1
  Data Type Conversion29/1 -> accel_r/1
  Data Type Conversion30/1 -> flags1/1
  In39/1 -> Data Type Conversion30/1
  In29/1 -> Data Type Conversion38/1
  Data Type Conversion38/1 -> speed_r/1
  Data Type Conversion37/1 -> speed_p/1
  In28/1 -> Data Type Conversion37/1
  In27/1 -> Data Type Conversion36/1
  Data Type Conversion36/1 -> speed_h/1
  Data Type Conversion35/1 -> speed_z/1
  In26/1 -> Data Type Conversion35/1
  Data Type Conversion39/1 -> flags2/1
  In30/1 -> Data Type Conversion39/1
  In25/1 -> Data Type Conversion34/1
  Data Type Conversion34/1 -> speed_y/1
  In21/1 -> Data Type Conversion20/1
  Data Type Conversion20/1 -> parent/1
  Data Type Conversion21/1 -> cfgFlags/1
  In22/1 -> Data Type Conversion21/1
  In23/1 -> Data Type Conversion32/1
  Data Type Conversion32/1 -> cfgModelId/1
  Data Type Conversion33/1 -> speed_x/1
  In24/1 -> Data Type Conversion33/1
  In42/1 -> Data Type Conversion41/1
  Data Type Conversion41/1 -> traveledDist/1
  Data Type Conversion40/1 -> system1/1
  In41/1 -> Data Type Conversion40/1
  Data Type Conversion42/1 -> spare_1/1
  In43/1 -> Data Type Conversion42/1
